simulink model "flatball_6dof_candp_wrk"  (R2021b)
settings: Solver=ode1be  StartTime=0.0  StopTime=30  FixedStep=1e-3  MaxStep=0.01  MinStep=0.01  RelTol=1e-3
values from neighbouring files (symbols this model uses):
  amb = evalin( 'base', 'amb')    [flatball_6dof_eqom.m]
  C = evalin( 'base', 'C')    [flatball_6dof_eqom.m]
  disc = evalin( 'base', 'disc')    [flatball_6dof_eqom.m]    (also in flatball_6dof_init.m = struct; flatball_init_disc_params.m = struct)
  k_launch_F_t_release = 0.60    (= 0.6)    [flatball_6dof_hucker_init.m]
  k_launch_Fx_kd = 2e-2    (= 0.02)    [flatball_6dof_hucker_init.m]
  k_launch_Fx_ki = 15    [flatball_6dof_hucker_init.m]
  k_launch_Fx_kp = 7.5    [flatball_6dof_hucker_init.m]
  k_launch_Fx_sat_hi = 150    [flatball_6dof_hucker_init.m]
  k_launch_Fx_sat_lo = -150    [flatball_6dof_hucker_init.m]
  k_launch_Fx_t_launch_begin = 0.50    (= 0.5)    [flatball_6dof_hucker_init.m]
  k_launch_Fx_t_launch_end = k_launch_F_t_release    (= 0.6)    [flatball_6dof_hucker_init.m]
  k_launch_Fy_kd = k_launch_Fx_kd    (= 0.02)    [flatball_6dof_hucker_init.m]
  k_launch_Fy_ki = k_launch_Fx_ki    (= 15)    [flatball_6dof_hucker_init.m]
  k_launch_Fy_kp = k_launch_Fx_kp    (= 7.5)    [flatball_6dof_hucker_init.m]
  k_launch_Fy_sat_hi = k_launch_Fx_sat_hi    (= 150)    [flatball_6dof_hucker_init.m]
  k_launch_Fy_sat_lo = k_launch_Fx_sat_lo    (= -150)    [flatball_6dof_hucker_init.m]
  k_launch_Fy_t_launch_begin = 0.50    (= 0.5)    [flatball_6dof_hucker_init.m]
  k_launch_Fy_t_launch_end = k_launch_F_t_release    (= 0.6)    [flatball_6dof_hucker_init.m]
  k_launch_Fz_kd = 2.5    [flatball_6dof_hucker_init.m]
  k_launch_Fz_ki = 50    [flatball_6dof_hucker_init.m]
  k_launch_Fz_kp = 20    [flatball_6dof_hucker_init.m]
  k_launch_Fz_sat_hi = 25    [flatball_6dof_hucker_init.m]
  k_launch_Fz_sat_lo = -25    [flatball_6dof_hucker_init.m]
  k_launch_Fz_t_launch_begin = 0.10    (= 0.1)    [flatball_6dof_hucker_init.m]
  k_launch_Fz_t_launch_end = k_launch_F_t_release    (= 0.6)    [flatball_6dof_hucker_init.m]
  k_launch_M_t_release = 0.60    (= 0.6)    [flatball_6dof_hucker_init.m]
  k_launch_Mx_kd = 0.125    [flatball_6dof_hucker_init.m]
  k_launch_Mx_ki = 1.125    [flatball_6dof_hucker_init.m]
  k_launch_Mx_kp = 3.5    [flatball_6dof_hucker_init.m]
  k_launch_Mx_sat_hi = 2.5    [flatball_6dof_hucker_init.m]
  k_launch_Mx_sat_lo = -2.5    [flatball_6dof_hucker_init.m]
  k_launch_Mx_t_launch_begin = 0.30    (= 0.3)    [flatball_6dof_hucker_init.m]
  k_launch_Mx_t_launch_end = k_launch_M_t_release    (= 0.6)    [flatball_6dof_hucker_init.m]
  k_launch_My_kd = 0.1125    [flatball_6dof_hucker_init.m]
  k_launch_My_ki = 5.5    [flatball_6dof_hucker_init.m]
  k_launch_My_kp = 4.25    [flatball_6dof_hucker_init.m]
  k_launch_My_sat_hi = 2.5    [flatball_6dof_hucker_init.m]
  k_launch_My_sat_lo = -2.5    [flatball_6dof_hucker_init.m]
  k_launch_My_t_launch_begin = 0.40    (= 0.4)    [flatball_6dof_hucker_init.m]
  k_launch_My_t_launch_end = k_launch_M_t_release    (= 0.6)    [flatball_6dof_hucker_init.m]
  k_launch_Mz_kd = 1e-8    (= 1e-08)    [flatball_6dof_hucker_init.m]
  k_launch_Mz_ki = 0.2575    [flatball_6dof_hucker_init.m]
  k_launch_Mz_kp = 0.25    [flatball_6dof_hucker_init.m]
  k_launch_Mz_sat_hi = 7.5    [flatball_6dof_hucker_init.m]
  k_launch_Mz_sat_lo = -7.5    [flatball_6dof_hucker_init.m]
  k_launch_Mz_t_launch_begin = 0.20    (= 0.2)    [flatball_6dof_hucker_init.m]
  k_launch_Mz_t_launch_end = k_launch_M_t_release    (= 0.6)    [flatball_6dof_hucker_init.m]
  XL_desired = [0 0 -45*C.IN2M, 5*C.DEG2RAD 5*C.DEG2RAD 0, 15 -3 0, 0 0 500*C.RPM2RADSEC]    [flatball_6dof_wrk.m]
undefined symbols (not defined in the file or in its folder): CandP, er, flatball, flatball_6dof_plnt_lib, huck, hucker_lib
libraries: slpidlib x6, simulink x5
(part 2 of 2)

== system flatball_6dof_candp_wrk/huck-er/Flaunch-ctrl/Subsystem ==
  Step2 : Step  Time=k_launch_Fx_t_launch_begin
  Step3 : Step  Time=k_launch_Fx_t_launch_end
  Sum3 : Sum  Inputs=+-
  Out1 : Outport
  wires:
  Step2/1 -> Sum3/1
  Step3/1 -> Sum3/2
  Sum3/1 -> Out1/1

== system flatball_6dof_candp_wrk/huck-er/Flaunch-ctrl/Subsystem1 ==
  Step4 : Step  Time=k_launch_Fy_t_launch_begin
  Step5 : Step  Time=k_launch_Fy_t_launch_end
  Sum4 : Sum  Inputs=+-
  Out1 : Outport
  wires:
  Step4/1 -> Sum4/1
  Step5/1 -> Sum4/2
  Sum4/1 -> Out1/1

== system flatball_6dof_candp_wrk/huck-er/Flaunch-ctrl/Subsystem2 ==
  Step : Step  Time=k_launch_Fz_t_launch_begin
  Step1 : Step  Time=k_launch_Fz_t_launch_end
  Sum4 : Sum  Inputs=+-
  Out1 : Outport
  wires:
  Step/1 -> Sum4/1
  Step1/1 -> Sum4/2
  Sum4/1 -> Out1/1

== system flatball_6dof_candp_wrk/huck-er/Mlaunch-ctrl/Subsystem ==
  Step5 : Step  Time=k_launch_Mx_t_launch_begin
  Step7 : Step  Time=k_launch_Mx_t_launch_end
  Sum3 : Sum  Inputs=+-
  Out1 : Outport
  wires:
  Step7/1 -> Sum3/2
  Sum3/1 -> Out1/1
  Step5/1 -> Sum3/1

== system flatball_6dof_candp_wrk/huck-er/Mlaunch-ctrl/Subsystem1 ==
  Step1 : Step  Time=k_launch_My_t_launch_begin
  Step4 : Step  Time=k_launch_My_t_launch_end
  Sum1 : Sum  Inputs=+-
  Out1 : Outport
  wires:
  Step4/1 -> Sum1/2
  Step1/1 -> Sum1/1
  Sum1/1 -> Out1/1

== system flatball_6dof_candp_wrk/huck-er/Mlaunch-ctrl/Subsystem2 ==
  Step2 : Step  Time=k_launch_Mz_t_launch_begin
  Step3 : Step  Time=k_launch_Mz_t_launch_end
  Sum2 : Sum  Inputs=+-
  Out1 : Outport
  wires:
  Step2/1 -> Sum2/1
  Step3/1 -> Sum2/2
  Sum2/1 -> Out1/1

== system flatball_6dof_candp_wrk/flatball-6dof-CandP/scopes/eml-6dof/lab ==
  dYdt : Inport
  Y : Inport  Port=2
  Compare To Constant : simulink/Logic and Bit Operations/Compare To Constant  relop=>=  const=0.0  OutDataTypeStr=boolean
  Demux : Demux  Outputs=[3 3 3 3]
  Demux1 : Demux  Outputs=[3 3 3 3]
  Selector : Selector  InputPortWidth=3  IndexOptions=Index vector (dialog)  Indices=[3]  OutputSizes=1
  Selector1 : Selector  InputPortWidth=3  IndexOptions=Index vector (dialog)  Indices=[1 2]  OutputSizes=1
  Stop Simulation : Stop
  TH1 : Scope
  TH1dot : Scope
  TH2dot : Scope
  TH2dotdot : Scope
  X1 : Scope
  X1dot : Scope
  X2dot : Scope
  X2dotdot : Scope
  wires:
  Compare To Constant/1 -> Stop Simulation/1
  Selector/1 -> Compare To Constant/1
  Selector1/1 -> TH1/1
  Y/1 -> Demux/1
  Demux/1 -> Selector/1, X1/1
  Demux/2 -> Selector1/1
  Demux/3 -> X2dot/1
  Demux/4 -> TH2dot/1
  dYdt/1 -> Demux1/1
  Demux1/1 -> X1dot/1
  Demux1/2 -> TH1dot/1
  Demux1/4 -> TH2dotdot/1
  Demux1/3 -> X2dotdot/1

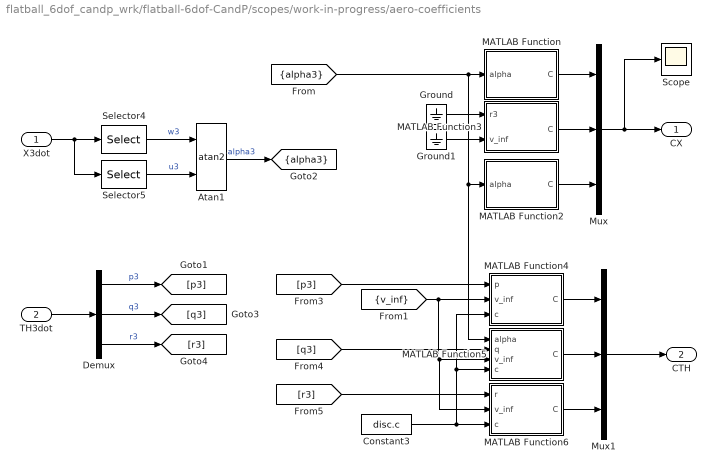
== system flatball_6dof_candp_wrk/flatball-6dof-CandP/scopes/work-in-progress/aero-coefficients ==
  X3dot : Inport
  TH3dot : Inport  Port=2
  Atan1 : Trigonometry  Operator=atan2
  Constant3 : Constant  Value=disc.c
  Demux : Demux  Outputs=3
  Ground : Ground
  Ground1 : Ground
  MATLAB Function : MATLAB Function  TreatAsAtomicUnit=on
  MATLAB Function2 : MATLAB Function  TreatAsAtomicUnit=on
  MATLAB Function3 : MATLAB Function  TreatAsAtomicUnit=on
  MATLAB Function4 : MATLAB Function  TreatAsAtomicUnit=on
  MATLAB Function5 : MATLAB Function  TreatAsAtomicUnit=on
  MATLAB Function6 : MATLAB Function  TreatAsAtomicUnit=on
  Mux : Mux  Inputs=3
  Mux1 : Mux  Inputs=3
  Scope : Scope
  Selector4 : Selector  InputPortWidth=3  IndexOptions=Index vector (dialog)  Indices=[3]  OutputSizes=1
  Selector5 : Selector  InputPortWidth=3  IndexOptions=Index vector (dialog)  Indices=[1]  OutputSizes=1
  CX : Outport
  CTH : Outport  Port=2
  tag scope: alpha3=scoped
  wires:
  Ground1/1 -> MATLAB Function3/2(v_inf)
  Ground/1 -> MATLAB Function3/1(r3)
  TH3dot/1 -> Demux/1
  [r3] -> MATLAB Function6/1(r)
  [q3] -> MATLAB Function5/2(q)
  [p3] -> MATLAB Function4/1(p)
  [v_inf] -> MATLAB Function4/2(v_inf), MATLAB Function5/3(v_inf), MATLAB Function6/2(v_inf)
  Constant3/1 -> MATLAB Function6/3(c), MATLAB Function5/4(c), MATLAB Function4/3(c)
  [alpha3] -> MATLAB Function/1(alpha), MATLAB Function5/1(alpha), MATLAB Function2/1(alpha)
  Mux1/1 -> CTH/1
  Mux/1 -> CX/1, Scope/1
  MATLAB Function4/1(C) -> Mux1/1
  MATLAB Function5/1(C) -> Mux1/2
  MATLAB Function6/1(C) -> Mux1/3
  MATLAB Function/1(C) -> Mux/1
  MATLAB Function2/1(C) -> Mux/3
  MATLAB Function3/1(C) -> Mux/2
  X3dot/1 -> Selector4/1, Selector5/1
  Demux/3 -> [r3]  "r3"
  Demux/2 -> [q3]  "q3"
  Demux/1 -> [p3]  "p3"
  Atan1/1 -> [alpha3]  "alpha3"
  Selector4/1 -> Atan1/1  "w3"
  Selector5/1 -> Atan1/2  "u3"

== system flatball_6dof_candp_wrk/flatball-6dof-CandP/scopes/work-in-progress/body-accelerations ==
  F2 : Inport
  M2 : Inport  Port=2
  Y : Inport  Port=3
  Constant1 : Constant  Value=disc.I
  Constant2 : Constant  Value=disc.m
  Constant3 : Constant  Value=disc.I ^ -1
  Product : Product  Multiplication=Matrix(*)
  Product1 : Product  Inputs=*/
  Product4 : Product  Inputs=3  Multiplication=Matrix(*)
  Product5 : Product  Multiplication=Matrix(*)
  Sum : Sum  Inputs=+-
  Sum1 : Sum  Inputs=+-
  TH2dot : Selector  InputPortWidth=12  IndexOptions=Index vector (dialog)  Indices=[10 11 12]  OutputSizes=1
  X2dot : Selector  InputPortWidth=12  IndexOptions=Index vector (dialog)  Indices=[7 8 9]  OutputSizes=1
  X2dotdot : Outport
  Th2dotdot : Outport  Port=2
  wires:
  TH2dot/1 -> Product4/3
  Constant1/1 -> Product4/2
  [w_tilde] -> Product4/1
  [w_tilde] -> Product/1
  Y/1 -> TH2dot/1, X2dot/1
  Product5/1 -> Th2dotdot/1
  Constant3/1 -> Product5/1
  Sum1/1 -> Product5/2
  Product4/1 -> Sum1/2
  M2/1 -> Sum1/1
  Sum/1 -> X2dotdot/1
  Product/1 -> Sum/2
  Product1/1 -> Sum/1
  Constant2/1 -> Product1/2
  F2/1 -> Product1/1
  X2dot/1 -> Product/2

== system flatball_6dof_candp_wrk/flatball-6dof-CandP/scopes/work-in-progress/body-forces-and-moments ==
  F4 : Inport
  M4 : Inport  Port=2
  Ground{,1..3} (4 alike) : Ground
  Mux : Mux  Inputs=3
  Mux1 : Mux  Inputs=3
  Product{,1..3} (4 alike) : Product  Multiplication=Matrix(*)
  Sum : Sum
  Transpose : Math  Operator=transpose  SaturateOnIntegerOverflow=on
  attitude-transformation : MATLAB Function  TreatAsAtomicUnit=on
  attitude-transformation1 : MATLAB Function  TreatAsAtomicUnit=on
  mg : Subsystem
  F2 : Outport
  M2 : Outport  Port=2
  wires:
  [Ta12] -> Product3/1
  [alpha3] -> Mux/2
  [beta2] -> Mux1/3
  mg/1(mg) -> Product3/2
  Sum/1 -> F2/1
  Product3/1 -> Sum/2
  Product2/1 -> M2/1
  Product1/1 -> Sum/1  "F2aero"
  [Ta42] -> Product2/1
  M4/1 -> Product2/2
  F4/1 -> Product1/2
  [Ta42] -> Product1/1
  Product/1 -> [Ta42]  "Ta42"
  attitude-transformation/1(T) -> Transpose/1  "Ta34"
  Transpose/1 -> Product/1  "Ta43"
  attitude-transformation1/1(T) -> Product/2  "Ta32"
  Ground2/1 -> Mux1/1
  Ground3/1 -> Mux1/2
  Mux1/1 -> attitude-transformation1/1(TH)
  Mux/1 -> attitude-transformation/1(TH)
  Ground/1 -> Mux/1
  Ground1/1 -> Mux/3

== system flatball_6dof_candp_wrk/flatball-6dof-CandP/scopes/work-in-progress/earth-reference ==
  Y : Inport
  Product : Product  Multiplication=Matrix(*)
  Product1 : Product  Multiplication=Matrix(*)
  TH1 : Selector  InputPortWidth=12  IndexOptions=Index vector (dialog)  Indices=[4 5 6]  OutputSizes=1
  TH2dot : Selector  InputPortWidth=12  IndexOptions=Index vector (dialog)  Indices=[10 11 12]  OutputSizes=1
  Transpose : Math  Operator=transpose  SaturateOnIntegerOverflow=on
  X2dot : Selector  InputPortWidth=12  IndexOptions=Index vector (dialog)  Indices=[7 8 9]  OutputSizes=1
  attitude-transformation : MATLAB Function  TreatAsAtomicUnit=on
  beta2 : Subsystem
  rate-transformation : MATLAB Function  TreatAsAtomicUnit=on
  v_inf : Subsystem
  w_tilde : Subsystem
  X1dot : Outport
  TH1dot : Outport  Port=2
  tag scope: Ta12=scoped
  wires:
  Transpose/1 -> [Ta12]
  [Ta21] -> Transpose/1
  Product1/1 -> TH1dot/1
  Product/1 -> X1dot/1
  [Tr21] -> Product1/1
  TH2dot/1 -> Product1/2  "TH2dot"
  X2dot/1 -> beta2/1(X2dot), v_inf/1(X2dot), w_tilde/1(X2dot), Product/2  "X2dot"
  [Ta21] -> Product/1
  rate-transformation/1(T) -> [Tr21]
  Y/1 -> TH2dot/1, X2dot/1, TH1/1
  attitude-transformation/1(T) -> [Ta21]
  TH1/1 -> rate-transformation/1(TH), attitude-transformation/1(TH)  "TH1"

== system flatball_6dof_candp_wrk/flatball-6dof-CandP/scopes/work-in-progress/eml-6dof ==
  Integrator4 : Integrator  InitialConditionSource=external
  MATLAB Function : MATLAB Function  TreatAsAtomicUnit=on
  f2302 : Constant  Value=[-0.90 -0.63 -0.91 -0.07 0.21 5.03 13.42 -0.41 0.001 -14.94 -1.48 54.25]
  lab : Subsystem
  wires:
  MATLAB Function/11(dydt) -> Integrator4/1
  MATLAB Function/9(alpha3) -> lab/9(alpha3)
  MATLAB Function/8(TH3dot) -> lab/8(TH3-dot)
  Integrator4/1 -> [X]  "X"
  MATLAB Function/1(X1) -> lab/1(X1)
  f2302/1 -> Integrator4/2, MATLAB Function/2(X0)
  [X] -> MATLAB Function/1(X)
  MATLAB Function/2(TH1) -> lab/2(TH1)
  MATLAB Function/5(X2dot) -> lab/5(X2-dot)
  MATLAB Function/6(TH2dot) -> lab/6(TH2-dot)
  MATLAB Function/4(TH1dot) -> lab/4(TH1-dot)
  MATLAB Function/10(beta2) -> lab/10(beta2)
  MATLAB Function/3(X1dot) -> lab/3(X1-dot)
  MATLAB Function/7(X3dot) -> lab/7(X3-dot)

== system flatball_6dof_candp_wrk/flatball-6dof-CandP/scopes/work-in-progress/lab ==
  dYdt : Inport
  Y : Inport  Port=2
  Compare To Constant : simulink/Logic and Bit Operations/Compare To Constant  relop=>=  const=0.0  OutDataTypeStr=boolean
  Demux : Demux  Outputs=[3 3 3 3]
  Demux1 : Demux  Outputs=[3 3 3 3]
  Gain : Gain  Gain=C.RAD2DEG
  Gain1 : Gain  Gain=C.RAD2DEG
  Scope1 : Scope
  Scope9 : Scope
  Selector : Selector  InputPortWidth=3  IndexOptions=Index vector (dialog)  Indices=[3]  OutputSizes=1
  Selector1 : Selector  InputPortWidth=3  IndexOptions=Index vector (dialog)  Indices=[1 2]  OutputSizes=1
  Stop Simulation : Stop
  TH1 : Scope
  TH1dot : Scope
  TH2dot : Scope
  TH2dotdot : Scope
  X1 : Scope
  X1dot : Scope
  X2dot : Scope
  X2dotdot : Scope
  wires:
  [beta2] -> Gain1/1
  [alpha3] -> Gain/1
  Demux1/3 -> X2dotdot/1
  Demux1/4 -> TH2dotdot/1
  Demux1/2 -> TH1dot/1
  Demux1/1 -> X1dot/1
  dYdt/1 -> Demux1/1
  Demux/4 -> TH2dot/1
  Demux/3 -> X2dot/1
  Demux/2 -> Selector1/1
  Demux/1 -> X1/1, Selector/1
  Y/1 -> Demux/1
  Selector1/1 -> TH1/1
  Gain1/1 -> Scope9/1
  Gain/1 -> Scope1/1
  Selector/1 -> Compare To Constant/1
  Compare To Constant/1 -> Stop Simulation/1

== system flatball_6dof_candp_wrk/flatball-6dof-CandP/scopes/work-in-progress/side-slip ==
  Y : Inport
  Ground : Ground
  Ground1 : Ground
  Mux : Mux  Inputs=3
  Product : Product  Multiplication=Matrix(*)
  Product1 : Product  Multiplication=Matrix(*)
  TH2dot : Selector  InputPortWidth=12  IndexOptions=Index vector (dialog)  Indices=[10 11 12]  OutputSizes=1
  Transpose : Math  Operator=transpose  SaturateOnIntegerOverflow=on
  X2dot : Selector  InputPortWidth=12  IndexOptions=Index vector (dialog)  Indices=[7 8 9]  OutputSizes=1
  attitude-transformation : MATLAB Function  TreatAsAtomicUnit=on
  X3dot : Outport
  TH3dot : Outport  Port=2
  wires:
  Transpose/1 -> [Ta23]  "Ta23"
  Ground1/1 -> Mux/2
  Ground/1 -> Mux/1
  attitude-transformation/1(T) -> Transpose/1  "Ta32"
  Mux/1 -> attitude-transformation/1(TH)
  [beta2] -> Mux/3
  Y/1 -> X2dot/1, TH2dot/1
  [Ta23] -> Product/1, Product1/1  "Ta23"
  X2dot/1 -> Product/2  "X2dot"
  TH2dot/1 -> Product1/2  "TH2dot"
  Product/1 -> X3dot/1
  Product1/1 -> TH3dot/1

== system flatball_6dof_candp_wrk/flatball-6dof-CandP/scopes/work-in-progress/wind-forces-and-moments ==
  CX : Inport
  CTH : Inport  Port=2
  Constant : Constant  Value=amb.rho / 2
  Constant1 : Constant  Value=disc.S
  Constant2 : Constant  Value=disc.c
  Demux : Demux  Outputs=3
  Gain : Gain  Gain=-1
  Gain1 : Gain  Gain=0
  Gain2 : Gain  Gain=-1
  Mux : Mux  Inputs=3
  Product1 : Product  Inputs=3
  Product2 : Product
  Product3 : Product
  Product4 : Product
  Square : Math  Operator=square  SaturateOnIntegerOverflow=on
  F4 : Outport
  M4 : Outport  Port=2
  wires:
  Constant2/1 -> Product1/3
  Product3/1 -> [qS]
  Square/1 -> Product4/2
  [v_inf] -> Square/1
  Product4/1 -> Product3/1  "q_inf"
  Constant/1 -> Product4/1
  Constant1/1 -> Product3/2
  Mux/1 -> Product2/1
  Gain2/1 -> Mux/3
  Gain/1 -> Mux/1
  Gain1/1 -> Mux/2
  Demux/3 -> Gain2/1
  Demux/2 -> Gain1/1
  Demux/1 -> Gain/1
  CX/1 -> Demux/1
  [qS] -> Product2/2, Product1/2
  CTH/1 -> Product1/1
  Product2/1 -> F4/1
  Product1/1 -> M4/1

== system flatball_6dof_candp_wrk/flatball-6dof-CandP/scopes/work-in-progress/body-forces-and-moments/mg ==
  Constant1 : Constant  Value=amb.g
  Constant2 : Constant  Value=disc.m
  Ground4 : Ground
  Ground5 : Ground
  Mux2 : Mux  Inputs=3
  Product4 : Product
  mg : Outport
  wires:
  Ground5/1 -> Mux2/2
  Mux2/1 -> Product4/2
  Constant2/1 -> Product4/1
  Ground4/1 -> Mux2/1
  Constant1/1 -> Mux2/3
  Product4/1 -> mg/1

== system flatball_6dof_candp_wrk/flatball-6dof-CandP/scopes/work-in-progress/earth-reference/beta2 ==
  X2dot : Inport
  Atan2 : Trigonometry  Operator=atan2
  Selector : Selector  InputPortWidth=3  IndexOptions=Index vector (dialog)  Indices=[2]  OutputSizes=1
  Selector3 : Selector  InputPortWidth=3  IndexOptions=Index vector (dialog)  Indices=[1]  OutputSizes=1
  tag scope: beta2=scoped
  wires:
  X2dot/1 -> Selector/1, Selector3/1
  Selector3/1 -> Atan2/2  "u2"
  Selector/1 -> Atan2/1  "v2"
  Atan2/1 -> [beta2]

== system flatball_6dof_candp_wrk/flatball-6dof-CandP/scopes/work-in-progress/earth-reference/v_inf ==
  X2dot : Inport
  Demux : Demux  Outputs=3
  Sqrt : Sqrt  SaturateOnIntegerOverflow=on
  Square : Math  Operator=square  SaturateOnIntegerOverflow=on
  Square1 : Math  Operator=square  SaturateOnIntegerOverflow=on
  Square2 : Math  Operator=square  SaturateOnIntegerOverflow=on
  Sum : Sum  Inputs=3
  tag scope: v_inf=scoped
  wires:
  Sqrt/1 -> [v_inf]
  Demux/2 -> Square1/1
  X2dot/1 -> Demux/1
  Demux/3 -> Square2/1
  Square/1 -> Sum/1
  Demux/1 -> Square/1
  Sum/1 -> Sqrt/1
  Square2/1 -> Sum/3
  Square1/1 -> Sum/2

== system flatball_6dof_candp_wrk/flatball-6dof-CandP/scopes/work-in-progress/earth-reference/w_tilde ==
  X2dot : Inport
  MATLAB Function : MATLAB Function  TreatAsAtomicUnit=on
  tag scope: w_tilde=scoped
  wires:
  X2dot/1 -> MATLAB Function/1(X2dot)
  MATLAB Function/1(w) -> [w_tilde]

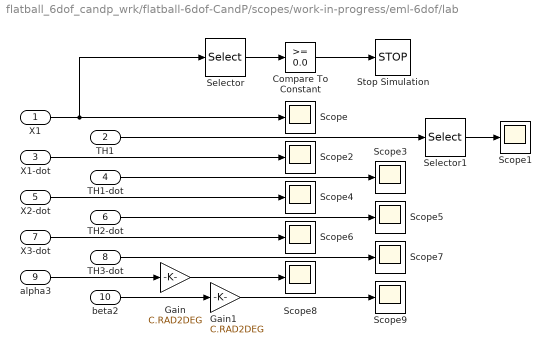
== system flatball_6dof_candp_wrk/flatball-6dof-CandP/scopes/work-in-progress/eml-6dof/lab ==
  X1 : Inport
  TH1 : Inport  Port=2
  X1-dot : Inport  Port=3
  TH1-dot : Inport  Port=4
  X2-dot : Inport  Port=5
  TH2-dot : Inport  Port=6
  X3-dot : Inport  Port=7
  TH3-dot : Inport  Port=8
  alpha3 : Inport  Port=9
  beta2 : Inport  Port=10
  Compare To Constant : simulink/Logic and Bit Operations/Compare To Constant  relop=>=  const=0.0  OutDataTypeStr=boolean
  Gain : Gain  Gain=C.RAD2DEG
  Gain1 : Gain  Gain=C.RAD2DEG
  Scope{,1..9} (10 alike) : Scope
  Selector : Selector  InputPortWidth=3  IndexOptions=Index vector (dialog)  Indices=[3]  OutputSizes=1
  Selector1 : Selector  InputPortWidth=3  IndexOptions=Index vector (dialog)  Indices=[1 2]  OutputSizes=1
  Stop Simulation : Stop
  wires:
  alpha3/1 -> Gain/1
  X1-dot/1 -> Scope2/1
  X3-dot/1 -> Scope6/1
  beta2/1 -> Gain1/1
  X1/1 -> Selector/1, Scope/1
  TH1/1 -> Selector1/1
  X2-dot/1 -> Scope4/1
  TH2-dot/1 -> Scope5/1
  TH1-dot/1 -> Scope3/1
  TH3-dot/1 -> Scope7/1
  Compare To Constant/1 -> Stop Simulation/1
  Selector/1 -> Compare To Constant/1
  Gain/1 -> Scope8/1
  Gain1/1 -> Scope9/1
  Selector1/1 -> Scope1/1

== matlab function flatball_6dof_candp_wrk/flatball-6dof-CandP/scopes/work-in-progress/aero-coefficients/MATLAB Function2 ==
  data: alpha input; C output
function C = Clift( alpha)
    CL0 = 0.13;
    CLa = 3.09;
    C = CL0 + CLa * alpha;

== matlab function flatball_6dof_candp_wrk/flatball-6dof-CandP/scopes/work-in-progress/aero-coefficients/MATLAB Function3 ==
  data: r3 input; C output; v_inf input
function C = Cside( r3, v_inf)
    C = -r3 * v_inf;

== matlab function flatball_6dof_candp_wrk/flatball-6dof-CandP/scopes/work-in-progress/aero-coefficients/MATLAB Function4 ==
  data: p input; C output; v_inf input; c input
function C = CL( p, v_inf, c)
    CLp = -1.30;
    C = CLp * p * c / (2 * v_inf);

== matlab function flatball_6dof_candp_wrk/flatball-6dof-CandP/scopes/work-in-progress/aero-coefficients/MATLAB Function5 ==
  data: alpha input; C output; q input; v_inf input; c input
function C = CM( alpha, q, v_inf, c)
    CM0 = -0.01;
    CMa = 0.057;
    CMq = -1.40;
    C = CM0 + CMa * alpha;
    C = C + CMq * q * c / (2 * v_inf);

== matlab function flatball_6dof_candp_wrk/flatball-6dof-CandP/scopes/work-in-progress/aero-coefficients/MATLAB Function6 ==
  data: r input; C output; v_inf input; c input
function C = CN( r, v_inf, c)
    CNr = -3e-2;
    C = CNr * r * c / (2 * v_inf);

== matlab function flatball_6dof_candp_wrk/flatball-6dof-CandP/scopes/work-in-progress/body-forces-and-moments/attitude-transformation ==
  data: T output; TH input
function T = Ta( TH) %(phi, theta, psi)
    phi = TH(1); theta = TH(2); psi = TH(3);
    T = [
        cos(theta)*cos(psi), sin(phi)*sin(theta)*cos(psi) - cos(phi)*sin(psi), cos(phi)*sin(theta)*cos(psi) + sin(phi)*sin(psi);
        cos(theta)*sin(psi), sin(phi)*sin(theta)*sin(psi) + cos(phi)*cos(psi), cos(phi)*sin(theta)*sin(psi) - sin(phi)*cos(psi);
        -sin(theta), -sin(phi)*cos(theta), cos(phi)*cos(theta)
        ];
end

== matlab function flatball_6dof_candp_wrk/flatball-6dof-CandP/scopes/work-in-progress/body-forces-and-moments/attitude-transformation1 ==
  data: T output; TH input
function T = Ta( TH) %(phi, theta, psi)
    phi = TH(1); theta = TH(2); psi = TH(3);
    T = [
        cos(theta)*cos(psi), sin(phi)*sin(theta)*cos(psi) - cos(phi)*sin(psi), cos(phi)*sin(theta)*cos(psi) + sin(phi)*sin(psi);
        cos(theta)*sin(psi), sin(phi)*sin(theta)*sin(psi) + cos(phi)*cos(psi), cos(phi)*sin(theta)*sin(psi) - sin(phi)*cos(psi);
        -sin(theta), -sin(phi)*cos(theta), cos(phi)*cos(theta)
        ];
end

== matlab function flatball_6dof_candp_wrk/flatball-6dof-CandP/scopes/work-in-progress/earth-reference/attitude-transformation ==
  data: T output; TH input
function T = Ta( TH) %(phi, theta, psi)
    phi = TH(1); theta = TH(2); psi = TH(3);
    T = [
        cos(theta)*cos(psi), sin(phi)*sin(theta)*cos(psi) - cos(phi)*sin(psi), cos(phi)*sin(theta)*cos(psi) + sin(phi)*sin(psi);
        cos(theta)*sin(psi), sin(phi)*sin(theta)*sin(psi) + cos(phi)*cos(psi), cos(phi)*sin(theta)*sin(psi) - sin(phi)*cos(psi);
        -sin(theta), -sin(phi)*cos(theta), cos(phi)*cos(theta)
        ];
end

== matlab function flatball_6dof_candp_wrk/flatball-6dof-CandP/scopes/work-in-progress/earth-reference/rate-transformation ==
  data: T output; TH input
function T = Tr( TH) %(phi, theta, psi)
    phi = TH(1); theta = TH(2); % psi = TH(3);
    T = [
        1, sin(phi)*tan(theta), cos(phi)*tan(theta);
        0, cos(phi), -sin(phi);
        0, sin(phi)*sec(theta), cos(phi)*sec(theta)
        ];
end

== matlab function flatball_6dof_candp_wrk/flatball-6dof-CandP/scopes/work-in-progress/earth-reference/w_tilde/MATLAB Function ==
  data: X2dot input; w output
function w = w_tilde( X2dot)
    p = X2dot(1); q = X2dot(2); r = X2dot(3);
    w = [
        0 -r q;
        r 0 -p;
        -q p 0
        ];

== matlab function flatball_6dof_candp_wrk/flatball-6dof-CandP/scopes/work-in-progress/eml-6dof/MATLAB Function ==
  data: X1 output; TH1 output; X1dot output; TH1dot output; X2dot output; TH2dot output; X3dot output; TH3dot output; alpha3 output; beta2 output; X input; dydt output; X0 input
function [X1, TH1, X1dot, TH1dot, X2dot, TH2dot, X3dot, TH3dot, alpha3, beta2, dydt] = flatball_6dof(X, X0)
%% define ambient conditions
amb.g = 9.7935; % m/s^2
amb.rho = 1.23; % Kg/m^3
%% define flatball (aka - frisbee)

% non-aerodynamic parameters
disc = struct;
disc.m = 0.175; % Kg
disc.I = [0.001219 0 0; 0 0.001219 0; 0 0 0.002352];
disc.c = 0.275;             % Reference chord length (m)
disc.S = pi*(0.275/2)^2;   % Reference area (m^2)

% define flatball aerodynamic properties
disc.alpha0 = -0.052;
disc.CD0 = 0.085;
disc.CDa = 3.30;
disc.CL0 = 0.13;
disc.CLa = 3.09;
disc.CLp = -1.30;
disc.CM0 = -0.01;
disc.CMa = 0.057;
disc.CMq = -1.40;
disc.CNr = -3e-2;

% NOTE: per simulation of a spin-stabilised sports disc
%       crowther & potts 2007
   
    % unpack state variables
    x = X(1); y = X(2); z = X(3);               % X1
    phi = X(4); theta = X(5); psi = X(6);       % TH1
    u = X(7); v = X(8); w = X(9);               % X2-dot
    p = X(10); q = X(11); r = X(12);            % TH2-dot
  
    % body reference variables
    X2dot = [u v w]';                           % X2-dot
    TH2dot = [p q r]';                          % TH2-dot

    v_inf = norm( X2dot);
    q_inf = (1/2) * amb.rho * v_inf^2;

    % calculate earth reference variables
    X1 = [x y z]';                              % X1
    TH1 = [phi theta psi]';                     % TH1

    Ta21 = Ta( TH1);
    Ta12 = Ta21';
    Tr21 = Tr( TH1);

    X1dot = Ta21 * X2dot;                       % X1-dot
    TH1dot = Tr21 * TH2dot;                     % TH1-dot

    % calculate zero sideslip variables
    u2 = X2dot(1); v2 = X2dot(2);
    beta2 = atan2( v2, u2);                     % sideslip angle
    
    Ta32 = Ta( [0 0 beta2]);
    Ta23 = Ta32';

    X3dot = Ta23 * X2dot;                       % X3-dot
    TH3dot = Ta23 * TH2dot;                     % TH3-dot

    % calculate aerodynamic coefficients
    u3 = X3dot(1); w3 = X3dot(3);
    p3 = TH3dot(1); q3 = TH3dot(2); r3 = TH3dot(3);

    alpha3 = atan2( w3, u3);                    % angle of attack
    
    CDrag = Cdrag_fcn( alpha3, disc);
    CSide = Cside_fcn( r3, v_inf);
    CLift = Clift_fcn( alpha3, disc);

    CL = CL_fcn( p3, v_inf, disc);
    CM = CM_fcn( alpha3, q3, v_inf, disc);
    CN = CN_fcn( r3, v_inf, disc);

    % calculate zero sideslip wind variables
    qS = q_inf * disc.S;
    qSc = qS * disc.c;
    mg = (disc.m .* [0 0 amb.g]');

    % calculate forces and moments
    Ta34 = Ta( [0 alpha3 0]);
    Ta43 = Ta34';
    
    F4 = qS * [-CDrag CSide -CLift]';           % F4
    M4 = qSc * [CL CM CN]';                     % M3

    F2aero = Ta43 * Ta32 * F4;
    F2 = F2aero + Ta12 * mg;                    % F2
    M2 = Ta43 * Ta32 * M4;                      % M2

    % calculate body accelerations
    w_tilde = [0 -r q; r 0 -p; -q p 0];
    X2dotdot = (F2 ./ disc.m ) - (w_tilde * X2dot);
    TH2dotdot = disc.I^-1 * (M2 - w_tilde * disc.I * TH2dot);

    dydt = [X1dot' TH1dot' X2dotdot' TH2dotdot']';
end

function T = Ta( TH) %(phi, theta, psi)
    phi = TH(1); theta = TH(2); psi = TH(3);
    T = [
        cos(theta)*cos(psi), sin(phi)*sin(theta)*cos(psi) - cos(phi)*sin(psi), cos(phi)*sin(theta)*cos(psi) + sin(phi)*sin(psi);
        cos(theta)*sin(psi), sin(phi)*sin(theta)*sin(psi) + cos(phi)*cos(psi), cos(phi)*sin(theta)*sin(psi) - sin(phi)*cos(psi);
        -sin(theta), -sin(phi)*cos(theta), cos(phi)*cos(theta)
        ];
end

function T = Tr( TH) %(phi, theta, psi)
    phi = TH(1); theta = TH(2); % psi = TH(3);
    T = [
        1, sin(phi)*tan(theta), cos(phi)*tan(theta);
        0, cos(phi), -sin(phi);
        0, sin(phi)*sec(theta), cos(phi)*sec(theta)
        ];
end

function C = Cdrag_fcn( alpha3, disc)
    C = disc.CD0 + disc.CDa * (alpha3 - disc.alpha0)^2;
end

function C = Clift_fcn( alpha3, disc)
    C = disc.CL0 + disc.CLa * alpha3;
end

function C = Cside_fcn( r3, vinf)
    C = -r3 * vinf * 0;                         % <-- 0 == no side force
end

function C = CL_fcn( p3, vinf, disc)
    C = disc.CLp * p3 * disc.c / (2 * vinf);
end

function C = CM_fcn( alpha, q3, vinf, disc)
    C = disc.CM0 + disc.CMa * alpha;
    C = C + (disc.CMq * q3 * disc.c / (2 * vinf));
end

function C = CN_fcn( r3, vinf, disc)
    C = disc.CNr * r3 * disc.c / (2 * vinf);
end

== matlab function flatball_6dof_candp_wrk/flatball-6dof-CandP/scopes/work-in-progress/side-slip/attitude-transformation ==
  data: T output; TH input
function T = Ta( TH) %(phi, theta, psi)
    phi = TH(1); theta = TH(2); psi = TH(3);
    T = [
        cos(theta)*cos(psi), sin(phi)*sin(theta)*cos(psi) - cos(phi)*sin(psi), cos(phi)*sin(theta)*cos(psi) + sin(phi)*sin(psi);
        cos(theta)*sin(psi), sin(phi)*sin(theta)*sin(psi) + cos(phi)*cos(psi), cos(phi)*sin(theta)*sin(psi) - sin(phi)*cos(psi);
        -sin(theta), -sin(phi)*cos(theta), cos(phi)*cos(theta)
        ];
end

== matlab function flatball_6dof_candp_wrk/flatball-6dof-CandP/body-forces-and-moments/attitude-transform ==
  data: T output; TH input
function T = Ta( TH)
% attitude transformation per Etkin and Reid 1995
phi = TH(1); theta = TH(2); psi = TH(3);
T = [
    cos(theta)*cos(psi), sin(phi)*sin(theta)*cos(psi) - cos(phi)*sin(psi), cos(phi)*sin(theta)*cos(psi) + sin(phi)*sin(psi);
    cos(theta)*sin(psi), sin(phi)*sin(theta)*sin(psi) + cos(phi)*cos(psi), cos(phi)*sin(theta)*sin(psi) - sin(phi)*cos(psi);
    -sin(theta), sin(phi)*cos(theta), cos(phi)*cos(theta)
    ];

== matlab function flatball_6dof_candp_wrk/flatball-6dof-CandP/earth-reference/attitude-transform ==
  data: T output; TH input
function T = Ta( TH)
% attitude transformation per Etkin and Reid 1995
phi = TH(1); theta = TH(2); psi = TH(3);
T = [
    cos(theta)*cos(psi), sin(phi)*sin(theta)*cos(psi) - cos(phi)*sin(psi), cos(phi)*sin(theta)*cos(psi) + sin(phi)*sin(psi);
    cos(theta)*sin(psi), sin(phi)*sin(theta)*sin(psi) + cos(phi)*cos(psi), cos(phi)*sin(theta)*sin(psi) - sin(phi)*cos(psi);
    -sin(theta), sin(phi)*cos(theta), cos(phi)*cos(theta)
    ];

== matlab function flatball_6dof_candp_wrk/flatball-6dof-CandP/earth-reference/rate-transform ==
  data: T output; TH input
function T = Tr( TH)
% euler angle rate transformation per Etkin and Reid 1995
phi = TH(1); theta = TH(2); % psi = TH(3);
T = [
    1, sin(phi)*tan(theta), cos(phi)*tan(theta);
    0, cos(phi), -sin(phi);
    0, sin(phi)*sec(theta), cos(phi)*sec(theta)
    ];

== matlab function flatball_6dof_candp_wrk/flatball-6dof-CandP/zero-side-slip-reference/attitude-transform ==
  data: T output; TH input
function T = Ta( TH)
% attitude transformation per Etkin and Reid 1995
phi = TH(1); theta = TH(2); psi = TH(3);
T = [
    cos(theta)*cos(psi), sin(phi)*sin(theta)*cos(psi) - cos(phi)*sin(psi), cos(phi)*sin(theta)*cos(psi) + sin(phi)*sin(psi);
    cos(theta)*sin(psi), sin(phi)*sin(theta)*sin(psi) + cos(phi)*cos(psi), cos(phi)*sin(theta)*sin(psi) - sin(phi)*cos(psi);
    -sin(theta), sin(phi)*cos(theta), cos(phi)*cos(theta)
    ];

== matlab function flatball_6dof_candp_wrk/flatball-6dof-CandP/body-accelerations/w-tilde ==
  data: w output; dTH2dt input
function w = w_tilde( dTH2dt)
    p = dTH2dt(1); q = dTH2dt( 2); r = dTH2dt(3);
    w = [0 -r q; r 0 -p; -q p 0];

== matlab function flatball_6dof_candp_wrk/flatball-6dof-CandP/scopes/eml-6dof/aero-coefficients ==
  data: X2dot input; alpha3 output; CX output; CTH output; X3dot input; TH3dot input
function [alpha3, CX, CTH] = flatball_6dof(X2dot, X3dot, TH3dot)
%% define ambient conditions
amb.g = 9.7935; % m/s^2
amb.rho = 1.23; % Kg/m^3
%% define flatball (aka - frisbee)

% non-aerodynamic parameters
disc = struct;
disc.m = 0.175; % Kg
disc.I = [0.001219 0 0; 0 0.001219 0; 0 0 0.002352];
disc.c = 0.275;             % Reference chord length (m)
disc.S = pi*(0.275/2)^2;   % Reference area (m^2)

% define flatball aerodynamic properties
disc.alpha0 = -0.052;
disc.CD0 = 0.085;
disc.CDa = 3.30;
disc.CL0 = 0.13;
disc.CLa = 3.09;
disc.CLp = -1.30;
disc.CM0 = -0.01;
disc.CMa = 0.057;
disc.CMq = -1.40;
disc.CNr = -3e-2;

    % calculate aerodynamic coefficients
    u3 = X3dot(1); w3 = X3dot(3);
    p3 = TH3dot(1); q3 = TH3dot(2); r3 = TH3dot(3);
    v_inf = norm( X2dot);

    alpha3 = atan2( w3, u3);                    % angle of attack
    
    CDrag = Cdrag_fcn( alpha3, disc);
    CSide = Cside_fcn( r3, v_inf);
    CLift = Clift_fcn( alpha3, disc);

    CL = CL_fcn( p3, v_inf, disc);
    CM = CM_fcn( alpha3, q3, v_inf, disc);
    CN = CN_fcn( r3, v_inf, disc);

    CX = [-CDrag CSide -CLift];
    CTH = [CL CM CN];
end

function C = Cdrag_fcn( alpha3, disc)
    C = disc.CD0 + disc.CDa * (alpha3 - disc.alpha0)^2;
end

function C = Clift_fcn( alpha3, disc)
    C = disc.CL0 + disc.CLa * alpha3;
end

function C = Cside_fcn( r3, vinf)
    C = -r3 * vinf * 0;                         % <-- 0 == no side force
end

function C = CL_fcn( p3, vinf, disc)
    C = disc.CLp * p3 * disc.c / (2 * vinf);
end

function C = CM_fcn( alpha, q3, vinf, disc)
    C = disc.CM0 + disc.CMa * alpha;
    C = C + (disc.CMq * q3 * disc.c / (2 * vinf));
end

function C = CN_fcn( r3, vinf, disc)
    C = disc.CNr * r3 * disc.c / (2 * vinf);
end

== matlab function flatball_6dof_candp_wrk/flatball-6dof-CandP/scopes/eml-6dof/body-accelerations ==
  data: X2dotdot output; TH2dotdot output; X2dot input; TH2dot input; F2 input; M2 input
function [X2dotdot, TH2dotdot] = flatball_6dof( X2dot, TH2dot, F2, M2)
%% define flatball (aka - frisbee)

% non-aerodynamic parameters
disc = struct;
disc.m = 0.175; % Kg
disc.I = [0.001219 0 0; 0 0.001219 0; 0 0 0.002352];
disc.c = 0.275;             % Reference chord length (m)
disc.S = pi*(0.275/2)^2;   % Reference area (m^2)

    % calculate body accelerations
    p = TH2dot(1); q = TH2dot( 2); r = TH2dot(3);
    w_tilde = [0 -r q; r 0 -p; -q p 0];
    X2dotdot = (F2 ./ disc.m ) - (w_tilde * X2dot);
    TH2dotdot = disc.I^-1 * (M2 - w_tilde * disc.I * TH2dot);
end

== matlab function flatball_6dof_candp_wrk/flatball-6dof-CandP/scopes/eml-6dof/body-force-and-moments ==
  data: F2 output; M2 output; alpha3 input; beta2 input; Ta12 input; F4 input; M4 input
function [F2, M2] = flatball_6dof( alpha3, beta2, Ta12, F4, M4)
%% define ambient conditions
amb.g = 9.7935; % m/s^2
%% define flatball (aka - frisbee)

% non-aerodynamic parameters
disc = struct;
disc.m = 0.175; % Kg

    % calculate forces and moments
    Ta32 = Ta( [0 0 beta2]);
    Ta34 = Ta( [0 alpha3 0]);
    Ta43 = Ta34';
    
    F2aero = Ta43 * Ta32 * F4;
    mg = (disc.m .* [0 0 amb.g]');
    F2 = F2aero + Ta12 * mg;                    % F2
    M2 = Ta43 * Ta32 * M4;                      % M2
end

function T = Ta( TH) %(phi, theta, psi)
    phi = TH(1); theta = TH(2); psi = TH(3);
    T = [
        cos(theta)*cos(psi), sin(phi)*sin(theta)*cos(psi) - cos(phi)*sin(psi), cos(phi)*sin(theta)*cos(psi) + sin(phi)*sin(psi);
        cos(theta)*sin(psi), sin(phi)*sin(theta)*sin(psi) + cos(phi)*cos(psi), cos(phi)*sin(theta)*sin(psi) - sin(phi)*cos(psi);
        -sin(theta), -sin(phi)*cos(theta), cos(phi)*cos(theta)
        ];
end

== matlab function flatball_6dof_candp_wrk/flatball-6dof-CandP/scopes/eml-6dof/earth-reference ==
  data: X1dot output; TH1dot output; Ta21 output; TH1 input; X2dot input; TH2dot input
function [X1dot, TH1dot, Ta21] = flatball_6dof(TH1, X2dot, TH2dot)
    %phi = TH1(1); theta = TH1(2); psi = TH1(3);
    %TH = [phi theta psi];
    Ta21 = Ta( TH1);
    Tr21 = Tr( TH1);

    X1dot = Ta21 * X2dot;                       % X1-dot
    TH1dot = Tr21 * TH2dot;                     % TH1-dotend
end

function T = Ta( TH) %(phi, theta, psi)
    phi = TH(1); theta = TH(2); psi = TH(3);
    T = [
        cos(theta)*cos(psi), sin(phi)*sin(theta)*cos(psi) - cos(phi)*sin(psi), cos(phi)*sin(theta)*cos(psi) + sin(phi)*sin(psi);
        cos(theta)*sin(psi), sin(phi)*sin(theta)*sin(psi) + cos(phi)*cos(psi), cos(phi)*sin(theta)*sin(psi) - sin(phi)*cos(psi);
        -sin(theta), -sin(phi)*cos(theta), cos(phi)*cos(theta)
        ];
end

function T = Tr( TH) %(phi, theta, psi)
    phi = TH(1); theta = TH(2); % psi = TH(3);
    T = [
        1, sin(phi)*tan(theta), cos(phi)*tan(theta);
        0, cos(phi), -sin(phi);
        0, sin(phi)*sec(theta), cos(phi)*sec(theta)
        ];
end

== matlab function flatball_6dof_candp_wrk/flatball-6dof-CandP/scopes/eml-6dof/side-slip-reference ==
  data: X3dot output; TH3dot output; beta2 output; X2dot input; TH2dot input
function [X3dot, TH3dot, beta2] = flatball_6dof(X2dot, TH2dot)
    % calculate zero sideslip variables
    u2 = X2dot(1); v2 = X2dot(2);
    beta2 = atan2( v2, u2);                     % sideslip angle
    
    Ta32 = Ta( [0 0 beta2]);
    Ta23 = Ta32';

    X3dot = Ta23 * X2dot;                       % X3-dot
    TH3dot = Ta23 * TH2dot;                     % TH3-dot
end

function T = Ta( TH) %(phi, theta, psi)
    phi = TH(1); theta = TH(2); psi = TH(3);
    T = [
        cos(theta)*cos(psi), sin(phi)*sin(theta)*cos(psi) - cos(phi)*sin(psi), cos(phi)*sin(theta)*cos(psi) + sin(phi)*sin(psi);
        cos(theta)*sin(psi), sin(phi)*sin(theta)*sin(psi) + cos(phi)*cos(psi), cos(phi)*sin(theta)*sin(psi) - sin(phi)*cos(psi);
        -sin(theta), -sin(phi)*cos(theta), cos(phi)*cos(theta)
        ];
end

== matlab function flatball_6dof_candp_wrk/flatball-6dof-CandP/scopes/eml-6dof/wind-force-and-moments ==
  data: X2dot input; F4 output; M4 output; CX input; CTH input
function [F4, M4] = flatball_6dof( X2dot, CX, CTH)
%% define ambient conditions
amb.g = 9.7935; % m/s^2
amb.rho = 1.23; % Kg/m^3
%% define flatball (aka - frisbee)

% non-aerodynamic parameters
disc = struct;
disc.m = 0.175; % Kg
disc.I = [0.001219 0 0; 0 0.001219 0; 0 0 0.002352];
disc.c = 0.275;             % Reference chord length (m)
disc.S = pi*(0.275/2)^2;   % Reference area (m^2)

% define flatball aerodynamic properties
disc.alpha0 = -0.052;
disc.CD0 = 0.085;
disc.CDa = 3.30;
disc.CL0 = 0.13;
disc.CLa = 3.09;
disc.CLp = -1.30;
disc.CM0 = -0.01;
disc.CMa = 0.057;
disc.CMq = -1.40;
disc.CNr = -3e-2;
    
    % calculate zero sideslip wind variables
    v_inf = norm( X2dot);
    q_inf = (1/2) * amb.rho * v_inf^2;
    qS = q_inf * disc.S;
    qSc = qS * disc.c;
    
    F4 = qS * CX';                              % F4
    M4 = qSc * CTH';                            % M3
end

== matlab function flatball_6dof_candp_wrk/flatball-6dof-CandP/scopes/work-in-progress/aero-coefficients/MATLAB Function ==
  data: alpha input; C output
function C = Cdrag( alpha)
    CD0 = 0.085;
    CDa = 3.30;
    alpha0 = -0.052;
    C = CD0 + CDa * (alpha - alpha0)^2;
